simulink model "MasterArbeit_EreignisgeneratorsNachTotzone"  (R2014a)
settings: Solver=ode45  StartTime=0  StopTime=25  RelTol=1e-3
StopFcn:
  | Evaluation
values from neighbouring files (symbols this model uses):
  Ereignis_Abtastzeit = 200    [DelayDensity_GeneticAlgorithm.m]
  Ereignisgenerator_Sampletime = 0.01    [DelayDensity_GeneticAlgorithm.m]
  Instanz = ResponstimeOfCase3(1:NumOfTask)/1000    [DelayDensity_FP_Simulation.m]    (also in LatenzInstanzErzeuger.m = zeros(1,Anzahl); LatenzInstanzErzeuger_Test.m = ResponstimeOfTask)
  Kd = 0.3    [DelayDensity_GeneticAlgorithm.m]
  Ki = 4    [DelayDensity_GeneticAlgorithm.m]
  Kp = 2    [DelayDensity_GeneticAlgorithm.m]
  NumOfTask = 40    [DelayDensityTestScript.m]    (also in DelayDensity_AConcrete_Generator.m = 2; DelayDensity_GeneticAlgorithm.m = 100; DelayDensity_OberschrankenTest_Script.m = 10; DelayDensity_OberschrankenTest_Script_5Tasks.m = 10)
  rho_Wert = 0.001    [DelayDensity_GeneticAlgorithm.m]
  sollwert = 15    [DelayDensityTestScript.m]    (also in DelayDensity_GeneticAlgorithm.m = 10)
  System_A = [0 1 0;0 0 1;0 -C/A -B/A]    [DelayDensity_GeneticAlgorithm.m]
  System_B = [0;0;1/A]    [DelayDensity_GeneticAlgorithm.m]
  System_S1 = [0;0;S1/A]    [DelayDensity_GeneticAlgorithm.m]
  System_S2 = [0;0;S2/A]    [DelayDensity_GeneticAlgorithm.m]
  time1 = StartTimeOfCase3(1:NumOfTask)/1000    [DelayDensity_FP_Simulation.m]    (also in LatenzInstanzErzeuger_Test.m = StartTimeOfTask)
  Totzone_Wert = 0.1    [DelayDensity_GeneticAlgorithm.m]
  Umax = 500    [DelayDensity_GeneticAlgorithm.m]
  V = -1/(System_C*inv(System_A-System_B*K)*System_B)    [DelayDensity_GeneticAlgorithm.m]
undefined symbols (not defined in the file or in its folder): K, magnitude
libraries: simulink x2
settings Model: Creator=shenc  LastModifiedBy=shenc

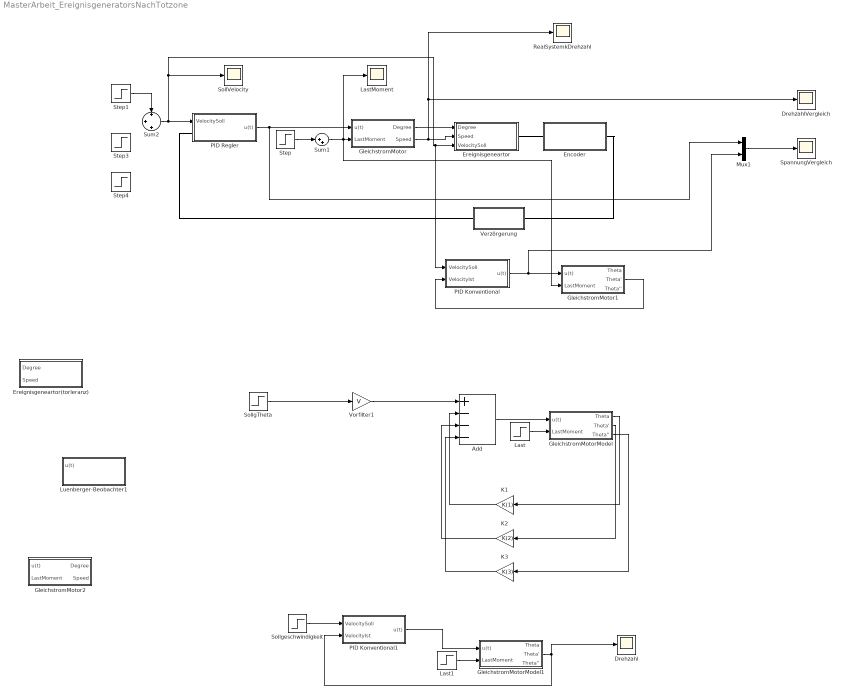
== system MasterArbeit_EreignisgeneratorsNachTotzone ==
  Add : Sum  Inputs=+---
  Drehzahl : Scope
      settings: ShowLegends=on  TimeRange=40  YMin=0  YMax=0.35  SaveName=Drehzahl1
  DrehzahlVergleich : Scope
      settings: ShowLegends=on  TimeRange=50  YMin=0  YMax=10  SaveName=Drehzahl
  Encoder : Subsystem
  Ereignisgeneartor : Subsystem
  Ereignisgeneartor(torleranz) : Subsystem
  GleichstromMotor : Subsystem
  GleichstromMotor1 : Subsystem
  GleichstromMotor2 : Subsystem
  GleichstromMotorModel : Subsystem
  GleichstromMotorModel1 : Subsystem
  K1 : Gain  Gain=K(1)
  K2 : Gain  Gain=K(2)
  K3 : Gain  Gain=K(3)
  Last : Step  Time=0  After=0  SampleTime=0
  Last1 : Step  Time=16  After=0.5  SampleTime=0
  LastMoment : Scope
      settings: ShowLegends=on  TimeRange=0.0001972721074048334  YMin=-4.75631690384965  YMax=-2.730597520382321  SaveName=ScopeData16
  Luenberger-Beobachter1 : Subsystem
  Mux1 : Mux  Inputs=2
  PID Konventional : Subsystem
  PID Konventional1 : Subsystem
  PID Regler : Subsystem
  RealSystemkDrehzahl : Scope
      settings: ShowLegends=on  TimeRange=24  YMin=9.783806343906511  YMax=15.78380634390651  SaveName=RealSystemDrehzahl
  SollVelocity : Scope
      settings: ShowLegends=on  TimeRange=0.0001972721074048334  YMin=-4.75631690384965  YMax=-2.730597520382321
  SollgTheta : Step  Time=0  After=5000  SampleTime=0
  Sollgeschwindigkeit : Step  Time=0  After=10  SampleTime=0
  SpannungVergleich : Scope
      settings: ShowLegends=on  TimeRange=0.0001972721074048334  YMin=-4.75631690384965  YMax=-2.730597520382321  SaveName=ScopeData4
  Step : Step  Time=15  After=0.3  SampleTime=0
  Step1 : Step  Time=0  After=sollwert  SampleTime=0
  Step3 : Step  Time=10  After=5  SampleTime=0
  Step4 : Step  Time=100  After=3  SampleTime=0
  Sum1 : Sum  Inputs=|++
  Sum2 : Sum  Inputs=+|+|+
  Verzörgerung : Subsystem
  Vorfilter1 : Gain  Gain=V
  wires:
  PID Regler/1(u(t)) -> Mux1/1, GleichstromMotor/1(u(t))
  Sum1/1 -> GleichstromMotor1/2(LastMoment), LastMoment/1, GleichstromMotor/2(LastMoment)
  Mux1/1 -> SpannungVergleich/1
  Sum2/1 -> PID Regler/1(VelocitySoll), PID Konventional/1(VelocitySoll), Ereignisgeneartor/3(VelocitySoll), SollVelocity/1
  Step1/1 -> Sum2/1
  GleichstromMotor/2(Speed) -> Ereignisgeneartor/2(Speed), DrehzahlVergleich/1, RealSystemkDrehzahl/1
  GleichstromMotor/1(Degree) -> Ereignisgeneartor/1(Degree)
  GleichstromMotor1/2(Theta') -> PID Konventional/2(VelocityIst)
  PID Konventional/1(u(t)) -> Mux1/2, GleichstromMotor1/1(u(t))
  Add/1 -> GleichstromMotorModel/1(u(t))
  GleichstromMotorModel/3(Theta'') -> K3/1
  K1/1 -> Add/2
  K2/1 -> Add/3
  K3/1 -> Add/4
  GleichstromMotorModel/1(Theta) -> K1/1
  GleichstromMotorModel/2(Theta') -> K2/1
  Last/1 -> GleichstromMotorModel/2(LastMoment)
  SollgTheta/1 -> Vorfilter1/1
  Vorfilter1/1 -> Add/1
  Sollgeschwindigkeit/1 -> PID Konventional1/1(VelocitySoll)
  PID Konventional1/1(u(t)) -> GleichstromMotorModel1/1(u(t))
  Last1/1 -> GleichstromMotorModel1/2(LastMoment)
  GleichstromMotorModel1/2(Theta') -> PID Konventional1/2(VelocityIst), Drehzahl/1
  Step/1 -> Sum1/1
  connections:
  Encoder/RConn1 -- Verzörgerung/LConn1
  Ereignisgeneartor/RConn1 -- Encoder/LConn1
  Verzörgerung/RConn1 -- PID Regler/LConn1

== system MasterArbeit_EreignisgeneratorsNachTotzone/Encoder ==
  Entity Sink : EntitySink
  Event-Based Entity Generator : EventBasedEntityGenerator  SignalEdgeType=Either
  Get Attribute : GetAttribute  AttributeName=Value|Speed  AttributeMissing=Error|Error  AttributeDefaultValue=1|1  AttributeTreatAsVector=1|1  AttributeSendTiming=After entity departure|After entity departure  StatNumberDeparted=on  EvaluatedDefaultAttributeValue={ [];[]}
      settings: OutputPortMap=o0,o1,o2
  Scope : Scope
      settings: SaveName=Event
  Scope1 : Scope
      settings: SaveName=Event1
  Scope2 : Scope
      settings: SaveName=Event2
  Set Attribute : SetAttribute  AttributeName=Value|Theta  AttributeFrom=Signal port|Signal port  AttributeValue=1|1  AttributeTreatAsVector=1|1  StatNumberDeparted=on  EvaluatedAttributeValue={ [];[]}
      settings: InputPortMap=u0,u1
  Degree : PMIOPort  Port=1  Side=Left
  V_Schatz : PMIOPort  Port=2  Side=Right
  wires:
  Get Attribute/3 -> Set Attribute/1, Scope2/1
  Set Attribute/1 -> Scope/1
  Get Attribute/1 -> Event-Based Entity Generator/1, Scope1/1
  Get Attribute/2 -> Set Attribute/2
  connections:
  Degree/RConn1 -- Get Attribute/LConn1
  Event-Based Entity Generator/RConn1 -- Set Attribute/LConn1
  Get Attribute/RConn1 -- Entity Sink/LConn1
  Set Attribute/RConn1 -- V_Schatz/RConn1

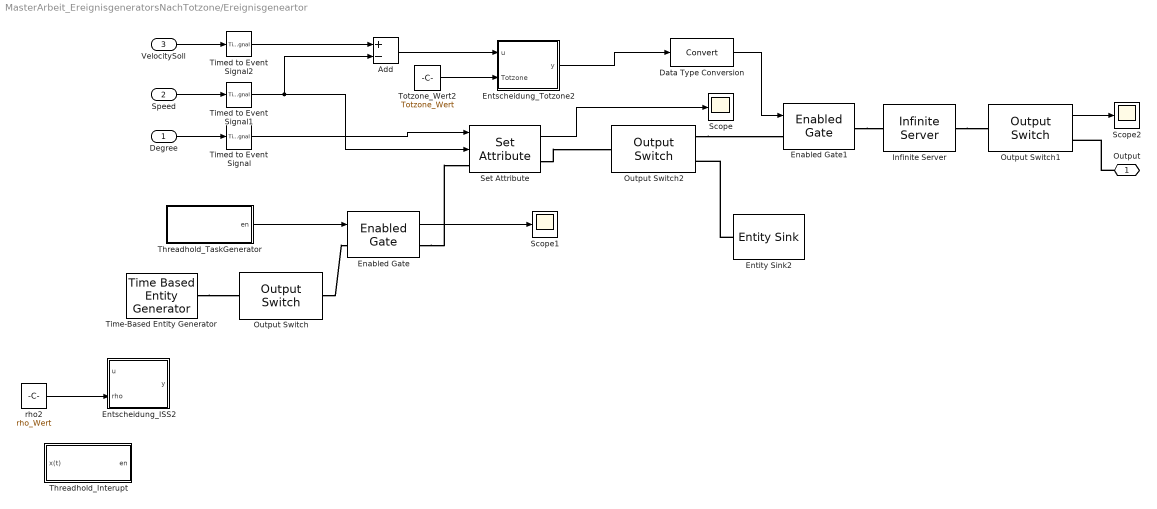
== system MasterArbeit_EreignisgeneratorsNachTotzone/Ereignisgeneartor ==
  Degree : Inport
  Speed : Inport  Port=2
  VelocitySoll : Inport  Port=3
  Add : Sum  Inputs=+-
  Data Type Conversion : DataTypeConversion
  Enabled Gate : EnabledGate  StatNumberDeparted=on
  Enabled Gate1 : EnabledGate
  Entity Sink2 : EntitySink
  Entscheidung_ISS2 : MATLAB Function  TreatAsAtomicUnit=on
  Entscheidung_Totzone2 : MATLAB Function  TreatAsAtomicUnit=on
  Infinite Server : InfiniteServer  ServiceTime=0.01
  Output Switch : OutputSwitch  NumberOutputPorts=1
  Output Switch1 : OutputSwitch  NumberOutputPorts=1  StatNumberDeparted=on
  Output Switch2 : OutputSwitch  NumberOutputPorts=2
  Scope : Scope
      settings: SaveName=ScopeData14
  Scope1 : Scope
      settings: SaveName=ScopeData19
  Scope2 : Scope
      settings: SaveName=Anzahl
  Set Attribute : SetAttribute  AttributeName=Value|Speed  AttributeFrom=Signal port|Signal port  AttributeValue=1|1  AttributeTreatAsVector=1|1  StatNumberDeparted=on  EvaluatedAttributeValue={ [];[]}
      settings: InputPortMap=u0,u1
  Threadhold_Interupt : Subsystem
  Threadhold_TaskGenerator : Subsystem
  Time-Based Entity Generator : TimeBasedEntityGenerator  Period=Ereignisgenerator_Sampletime
  Timed to Event Signal : TimedToEventSignal
  Timed to Event Signal1 : TimedToEventSignal
  Timed to Event Signal2 : TimedToEventSignal
  Totzone_Wert2 : Constant  Value=Totzone_Wert
  rho2 : Constant  Value=rho_Wert
  Output : PMIOPort  Port=1  Side=Right
  wires:
  Timed to Event Signal/1 -> Set Attribute/1
  Degree/1 -> Timed to Event Signal/1
  Speed/1 -> Timed to Event Signal1/1
  Timed to Event Signal1/1 -> Add/2, Set Attribute/2
  Data Type Conversion/1 -> Enabled Gate1/1
  VelocitySoll/1 -> Timed to Event Signal2/1
  Add/1 -> Entscheidung_Totzone2/1(u)
  Timed to Event Signal2/1 -> Add/1
  Set Attribute/1 -> Scope/1
  Enabled Gate/1 -> Scope1/1
  Output Switch1/1 -> Scope2/1
  Entscheidung_Totzone2/1(y) -> Data Type Conversion/1
  Threadhold_TaskGenerator/1(en) -> Enabled Gate/1
  rho2/1 -> Entscheidung_ISS2/2(rho)
  Totzone_Wert2/1 -> Entscheidung_Totzone2/2(Totzone)
  connections:
  Time-Based Entity Generator/RConn1 -- Output Switch/LConn1
  Output Switch/RConn1 -- Enabled Gate/LConn1
  Enabled Gate/RConn1 -- Set Attribute/LConn1
  Infinite Server/RConn1 -- Output Switch1/LConn1
  Output/RConn1 -- Output Switch1/RConn1
  Set Attribute/RConn1 -- Output Switch2/LConn1
  Entity Sink2/LConn1 -- Output Switch2/RConn2
  Output Switch2/RConn1 -- Enabled Gate1/LConn1
  Enabled Gate1/RConn1 -- Infinite Server/LConn1

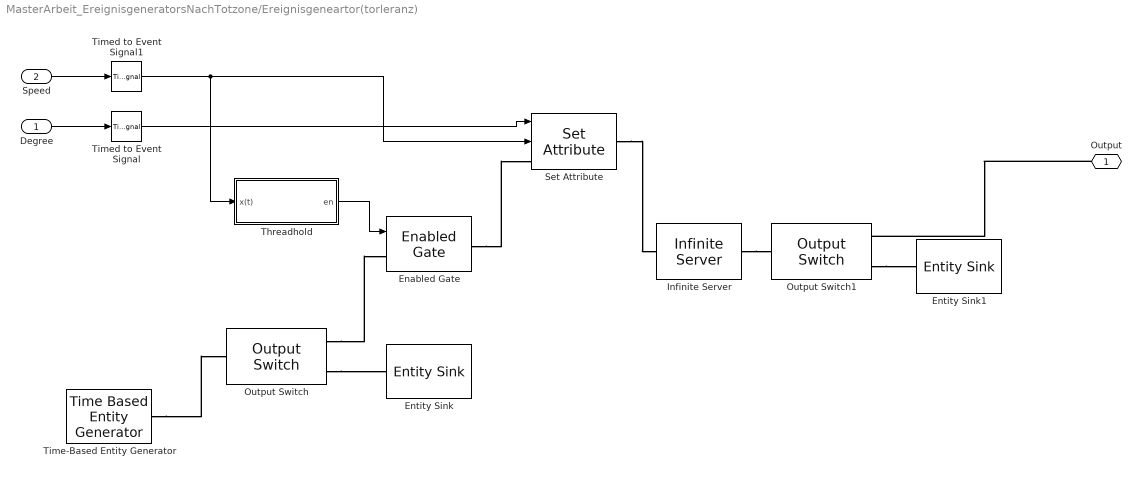
== system MasterArbeit_EreignisgeneratorsNachTotzone/Ereignisgeneartor(torleranz) ==
  Degree : Inport
  Speed : Inport  Port=2
  Enabled Gate : EnabledGate
  Entity Sink : EntitySink
  Entity Sink1 : EntitySink
  Infinite Server : InfiniteServer  ServiceTime=0.01
  Output Switch : OutputSwitch  NumberOutputPorts=2
  Output Switch1 : OutputSwitch  NumberOutputPorts=2
  Set Attribute : SetAttribute  AttributeName=Value|Speed  AttributeFrom=Signal port|Signal port  AttributeValue=1|1  AttributeTreatAsVector=1|1  EvaluatedAttributeValue={ [];[]}
      settings: InputPortMap=u0,u1
  Threadhold : Subsystem
  Time-Based Entity Generator : TimeBasedEntityGenerator  Period=Ereignisgenerator_Sampletime
  Timed to Event Signal : TimedToEventSignal
  Timed to Event Signal1 : TimedToEventSignal
  Output : PMIOPort  Port=1  Side=Right
  wires:
  Threadhold/1(en) -> Enabled Gate/1
  Timed to Event Signal/1 -> Set Attribute/1
  Degree/1 -> Timed to Event Signal/1
  Speed/1 -> Timed to Event Signal1/1
  Timed to Event Signal1/1 -> Threadhold/1(x(t)), Set Attribute/2
  connections:
  Time-Based Entity Generator/RConn1 -- Output Switch/LConn1
  Output Switch/RConn2 -- Entity Sink/LConn1
  Output Switch/RConn1 -- Enabled Gate/LConn1
  Set Attribute/RConn1 -- Infinite Server/LConn1
  Enabled Gate/RConn1 -- Set Attribute/LConn1
  Infinite Server/RConn1 -- Output Switch1/LConn1
  Output/RConn1 -- Output Switch1/RConn1
  Output Switch1/RConn2 -- Entity Sink1/LConn1

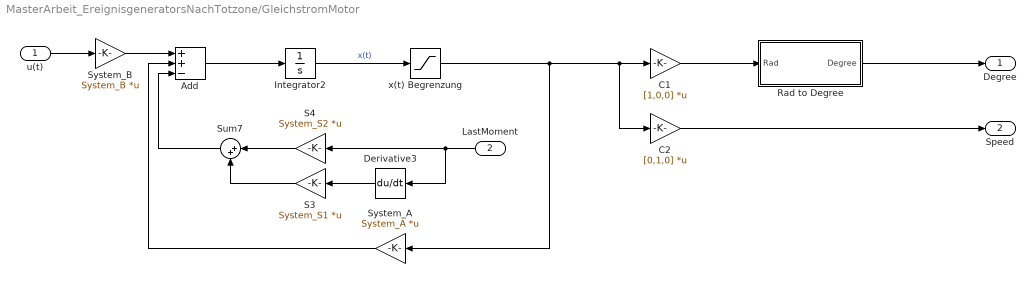
== system MasterArbeit_EreignisgeneratorsNachTotzone/GleichstromMotor ==
  u(t) : Inport
  LastMoment : Inport  Port=2
  Add : Sum  Inputs=++-
  C1 : Gain  Gain=[1,0,0]  Multiplication=Matrix(K*u)
  C2 : Gain  Gain=[0,1,0]  Multiplication=Matrix(K*u)
  Derivative3 : Derivative
  Integrator2 : Integrator
  Rad to Degree : Subsystem
  S3 : Gain  Gain=System_S1  Multiplication=Matrix(K*u)
  S4 : Gain  Gain=System_S2  Multiplication=Matrix(K*u)
  Sum7 : Sum  Inputs=|++
  System_A : Gain  Gain=System_A  Multiplication=Matrix(K*u)
  System_B : Gain  Gain=System_B  Multiplication=Matrix(K*u)
  x(t) Begrenzung : Saturate  UpperLimit=[inf,inf,20]  LowerLimit=-50
  Degree : Outport
  Speed : Outport  Port=2
  wires:
  Derivative3/1 -> S3/1
  S4/1 -> Sum7/1
  S3/1 -> Sum7/2
  u(t)/1 -> System_B/1
  C1/1 -> Rad to Degree/1(Rad)
  Integrator2/1 -> x(t) Begrenzung/1  "x(t)"
  Rad to Degree/1(Degree) -> Degree/1
  LastMoment/1 -> Derivative3/1, S4/1
  C2/1 -> Speed/1
  x(t) Begrenzung/1 -> C2/1, C1/1, System_A/1
  System_B/1 -> Add/1
  System_A/1 -> Add/2
  Sum7/1 -> Add/3
  Add/1 -> Integrator2/1

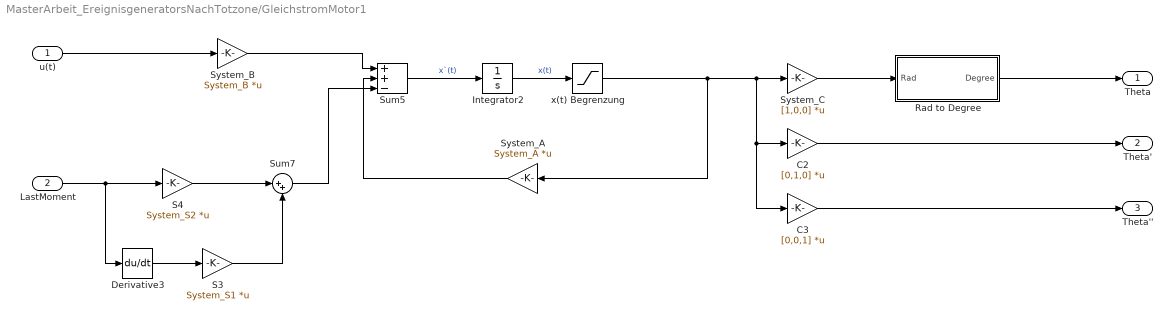
== system MasterArbeit_EreignisgeneratorsNachTotzone/GleichstromMotor1 ==
  u(t) : Inport
  LastMoment : Inport  Port=2
  C2 : Gain  Gain=[0,1,0]  Multiplication=Matrix(K*u)
  C3 : Gain  Gain=[0,0,1]  Multiplication=Matrix(K*u)
  Derivative3 : Derivative
  Integrator2 : Integrator
  Rad to Degree : Subsystem
  S3 : Gain  Gain=System_S1  Multiplication=Matrix(K*u)
  S4 : Gain  Gain=System_S2  Multiplication=Matrix(K*u)
  Sum5 : Sum  Inputs=+|+|-
  Sum7 : Sum  Inputs=|++
  System_A : Gain  Gain=System_A  Multiplication=Matrix(K*u)
  System_B : Gain  Gain=System_B  Multiplication=Matrix(K*u)
  System_C : Gain  Gain=[1,0,0]  Multiplication=Matrix(K*u)
  x(t) Begrenzung : Saturate  UpperLimit=[inf,inf,20]  LowerLimit=-50
  Theta : Outport
  Theta' : Outport  Port=2
  Theta'' : Outport  Port=3
  wires:
  Sum5/1 -> Integrator2/1  "x`(t)"
  System_A/1 -> Sum5/2
  u(t)/1 -> System_B/1
  System_B/1 -> Sum5/1
  System_C/1 -> Rad to Degree/1(Rad)
  Integrator2/1 -> x(t) Begrenzung/1  "x(t)"
  Rad to Degree/1(Degree) -> Theta/1
  C2/1 -> Theta'/1
  C3/1 -> Theta''/1
  x(t) Begrenzung/1 -> C3/1, C2/1, System_C/1, System_A/1
  LastMoment/1 -> Derivative3/1, S4/1
  S4/1 -> Sum7/1
  Derivative3/1 -> S3/1
  S3/1 -> Sum7/2
  Sum7/1 -> Sum5/3

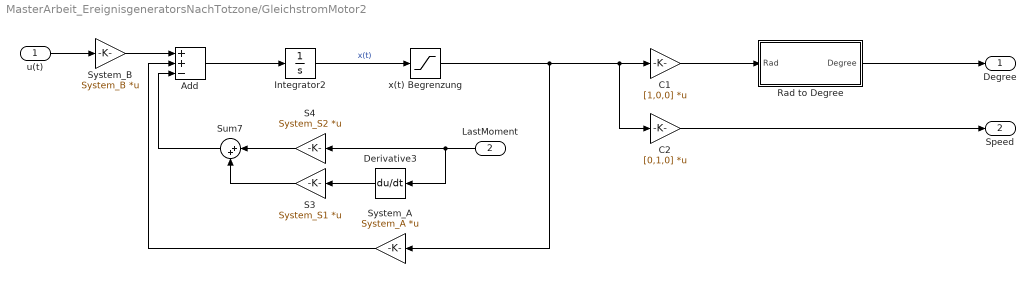
== system MasterArbeit_EreignisgeneratorsNachTotzone/GleichstromMotor2 ==
  u(t) : Inport
  LastMoment : Inport  Port=2
  Add : Sum  Inputs=++-
  C1 : Gain  Gain=[1,0,0]  Multiplication=Matrix(K*u)
  C2 : Gain  Gain=[0,1,0]  Multiplication=Matrix(K*u)
  Derivative3 : Derivative
  Integrator2 : Integrator
  Rad to Degree : Subsystem
  S3 : Gain  Gain=System_S1  Multiplication=Matrix(K*u)
  S4 : Gain  Gain=System_S2  Multiplication=Matrix(K*u)
  Sum7 : Sum  Inputs=|++
  System_A : Gain  Gain=System_A  Multiplication=Matrix(K*u)
  System_B : Gain  Gain=System_B  Multiplication=Matrix(K*u)
  x(t) Begrenzung : Saturate  UpperLimit=[inf,inf,20]  LowerLimit=-50
  Degree : Outport
  Speed : Outport  Port=2
  wires:
  Derivative3/1 -> S3/1
  S4/1 -> Sum7/1
  S3/1 -> Sum7/2
  u(t)/1 -> System_B/1
  C1/1 -> Rad to Degree/1(Rad)
  Integrator2/1 -> x(t) Begrenzung/1  "x(t)"
  Rad to Degree/1(Degree) -> Degree/1
  LastMoment/1 -> Derivative3/1, S4/1
  C2/1 -> Speed/1
  x(t) Begrenzung/1 -> C2/1, C1/1, System_A/1
  System_B/1 -> Add/1
  System_A/1 -> Add/2
  Sum7/1 -> Add/3
  Add/1 -> Integrator2/1

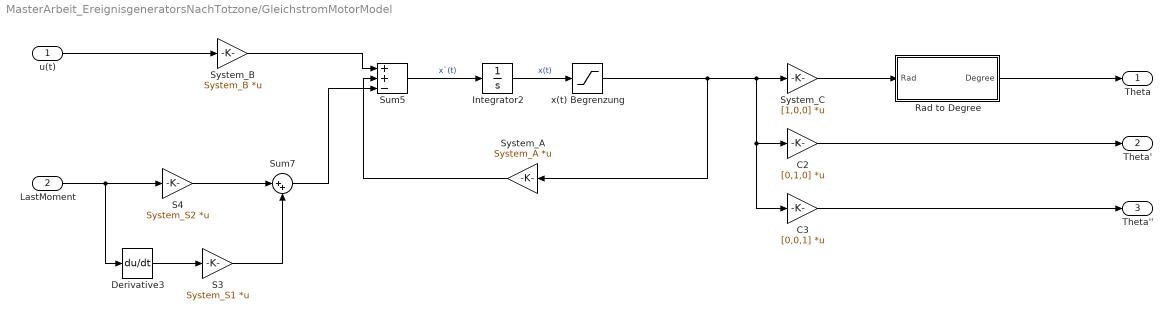
== system MasterArbeit_EreignisgeneratorsNachTotzone/GleichstromMotorModel ==
  u(t) : Inport
  LastMoment : Inport  Port=2
  C2 : Gain  Gain=[0,1,0]  Multiplication=Matrix(K*u)
  C3 : Gain  Gain=[0,0,1]  Multiplication=Matrix(K*u)
  Derivative3 : Derivative
  Integrator2 : Integrator
  Rad to Degree : Subsystem
  S3 : Gain  Gain=System_S1  Multiplication=Matrix(K*u)
  S4 : Gain  Gain=System_S2  Multiplication=Matrix(K*u)
  Sum5 : Sum  Inputs=+|+|-
  Sum7 : Sum  Inputs=|++
  System_A : Gain  Gain=System_A  Multiplication=Matrix(K*u)
  System_B : Gain  Gain=System_B  Multiplication=Matrix(K*u)
  System_C : Gain  Gain=[1,0,0]  Multiplication=Matrix(K*u)
  x(t) Begrenzung : Saturate  UpperLimit=[inf,inf,20]  LowerLimit=-50
  Theta : Outport
  Theta' : Outport  Port=2
  Theta'' : Outport  Port=3
  wires:
  Sum5/1 -> Integrator2/1  "x`(t)"
  System_A/1 -> Sum5/2
  u(t)/1 -> System_B/1
  System_B/1 -> Sum5/1
  System_C/1 -> Rad to Degree/1(Rad)
  Integrator2/1 -> x(t) Begrenzung/1  "x(t)"
  C2/1 -> Theta'/1
  C3/1 -> Theta''/1
  x(t) Begrenzung/1 -> C3/1, C2/1, System_C/1, System_A/1
  LastMoment/1 -> Derivative3/1, S4/1
  S4/1 -> Sum7/1
  Derivative3/1 -> S3/1
  S3/1 -> Sum7/2
  Sum7/1 -> Sum5/3
  Rad to Degree/1(Degree) -> Theta/1

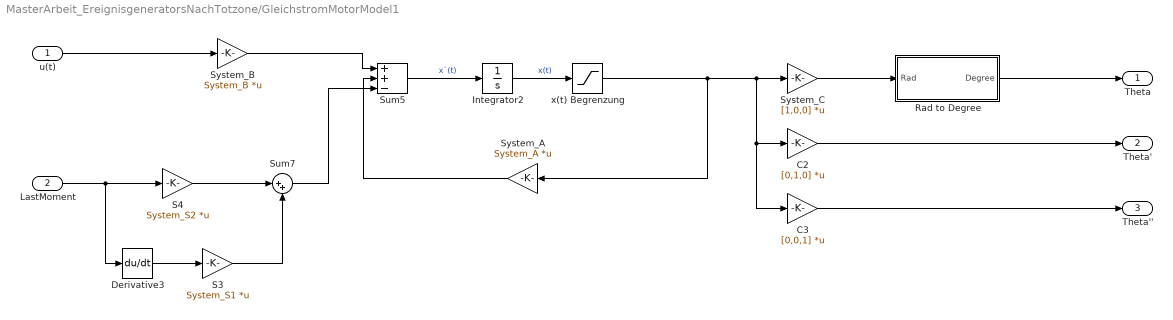
== system MasterArbeit_EreignisgeneratorsNachTotzone/GleichstromMotorModel1 ==
  u(t) : Inport
  LastMoment : Inport  Port=2
  C2 : Gain  Gain=[0,1,0]  Multiplication=Matrix(K*u)
  C3 : Gain  Gain=[0,0,1]  Multiplication=Matrix(K*u)
  Derivative3 : Derivative
  Integrator2 : Integrator
  Rad to Degree : Subsystem
  S3 : Gain  Gain=System_S1  Multiplication=Matrix(K*u)
  S4 : Gain  Gain=System_S2  Multiplication=Matrix(K*u)
  Sum5 : Sum  Inputs=+|+|-
  Sum7 : Sum  Inputs=|++
  System_A : Gain  Gain=System_A  Multiplication=Matrix(K*u)
  System_B : Gain  Gain=System_B  Multiplication=Matrix(K*u)
  System_C : Gain  Gain=[1,0,0]  Multiplication=Matrix(K*u)
  x(t) Begrenzung : Saturate  UpperLimit=[inf,inf,20]  LowerLimit=-50
  Theta : Outport
  Theta' : Outport  Port=2
  Theta'' : Outport  Port=3
  wires:
  Sum5/1 -> Integrator2/1  "x`(t)"
  System_A/1 -> Sum5/2
  u(t)/1 -> System_B/1
  System_B/1 -> Sum5/1
  System_C/1 -> Rad to Degree/1(Rad)
  Integrator2/1 -> x(t) Begrenzung/1  "x(t)"
  C2/1 -> Theta'/1
  C3/1 -> Theta''/1
  x(t) Begrenzung/1 -> C3/1, C2/1, System_C/1, System_A/1
  LastMoment/1 -> Derivative3/1, S4/1
  S4/1 -> Sum7/1
  Derivative3/1 -> S3/1
  S3/1 -> Sum7/2
  Sum7/1 -> Sum5/3
  Rad to Degree/1(Degree) -> Theta/1

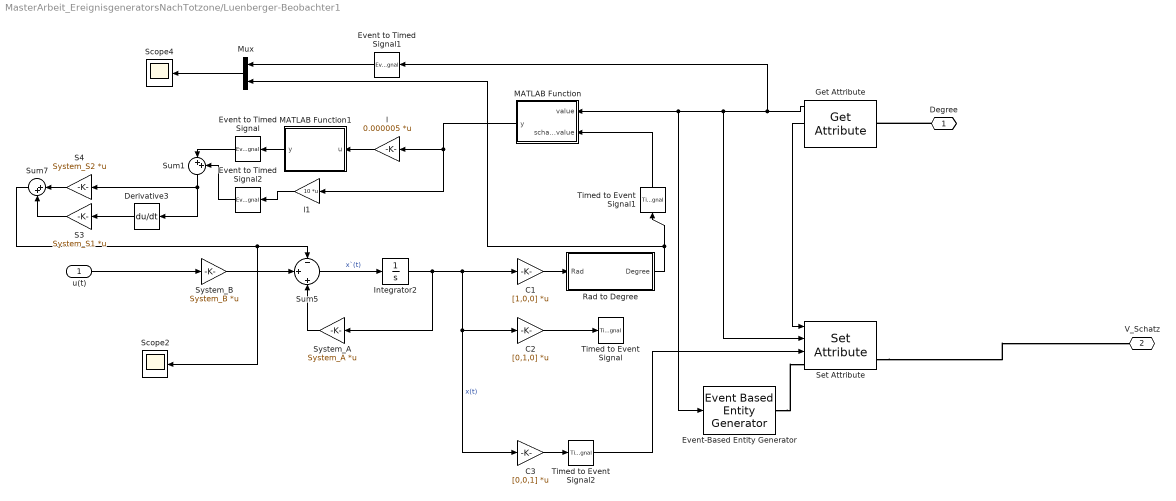
== system MasterArbeit_EreignisgeneratorsNachTotzone/Luenberger-Beobachter1 ==
  u(t) : Inport
  C1 : Gain  Gain=[1,0,0]  Multiplication=Matrix(K*u)
  C2 : Gain  Gain=[0,1,0]  Multiplication=Matrix(K*u)
  C3 : Gain  Gain=[0,0,1]  Multiplication=Matrix(K*u)
  Derivative3 : Derivative
  Event to Timed Signal : EventToTimedSignal
  Event to Timed Signal1 : EventToTimedSignal
  Event to Timed Signal2 : EventToTimedSignal
  Event-Based Entity Generator : EventBasedEntityGenerator  SignalEdgeType=Either
  Get Attribute : GetAttribute  AttributeName=Value|Speed  AttributeMissing=Error|Error  AttributeDefaultValue=1|1  AttributeTreatAsVector=1|1  AttributeSendTiming=After entity departure|After entity departure  EvaluatedDefaultAttributeValue={ [];[]}
      settings: OutputPortMap=o1,o2
  Integrator2 : Integrator
  MATLAB Function : MATLAB Function  TreatAsAtomicUnit=on
  MATLAB Function1 : MATLAB Function  TreatAsAtomicUnit=on
  Mux : Mux  Inputs=2
  Rad to Degree : Subsystem
  S3 : Gain  Gain=System_S1  Multiplication=Matrix(K*u)
  S4 : Gain  Gain=System_S2  Multiplication=Matrix(K*u)
  Scope2 : Scope
      settings: ShowLegends=on  TimeRange=10  YMin=0  YMax=275  SaveName=ScopeData15
  Scope4 : Scope
      settings: ShowLegends=on  TimeRange=10  YMin=0  YMax=275  SaveName=ScopeData13
  Set Attribute : SetAttribute  AttributeName=Value|Theta|Beschleunigung  AttributeFrom=Signal port|Signal port|Signal port  AttributeValue=1|1|1  AttributeTreatAsVector=1|1|1  StatNumberDeparted=on  EvaluatedAttributeValue={ [];[];[]}
      settings: InputPortMap=u0,u1,u2
  Sum1 : Sum  Inputs=|++
  Sum5 : Sum  Inputs=-|+|+
  Sum7 : Sum  Inputs=|++
  System_A : Gain  Gain=System_A  Multiplication=Matrix(K*u)
  System_B : Gain  Gain=System_B  Multiplication=Matrix(K*u)
  Timed to Event Signal : TimedToEventSignal
  Timed to Event Signal1 : TimedToEventSignal
  Timed to Event Signal2 : TimedToEventSignal
  l : Gain  Gain=0.000005  Multiplication=Matrix(K*u)
  l1 : Gain  Gain=10  Multiplication=Matrix(K*u)
  Degree : PMIOPort  Port=1  Side=Left
  V_Schatz : PMIOPort  Port=2  Side=Right
  wires:
  C1/1 -> Rad to Degree/1(Rad)
  Integrator2/1 -> System_A/1, C2/1, C3/1, C1/1  "x(t)"
  System_B/1 -> Sum5/2
  System_A/1 -> Sum5/3
  C3/1 -> Timed to Event Signal2/1
  Sum5/1 -> Integrator2/1  "x`(t)"
  Get Attribute/1 -> Event to Timed Signal1/1, Set Attribute/2, MATLAB Function/1(value), Event-Based Entity Generator/1
  Timed to Event Signal2/1 -> Set Attribute/3
  Mux/1 -> Scope4/1
  Rad to Degree/1(Degree) -> Mux/2, Timed to Event Signal1/1
  Timed to Event Signal1/1 -> MATLAB Function/2(schatzvalue)
  Event to Timed Signal1/1 -> Mux/1
  u(t)/1 -> System_B/1
  Derivative3/1 -> S3/1
  S4/1 -> Sum7/1
  S3/1 -> Sum7/2
  Sum7/1 -> Sum5/1, Scope2/1
  l/1 -> MATLAB Function1/1(u)
  MATLAB Function1/1(y) -> Event to Timed Signal/1
  MATLAB Function/1(y) -> l1/1, l/1
  C2/1 -> Timed to Event Signal/1
  Sum1/1 -> S4/1, Derivative3/1
  l1/1 -> Event to Timed Signal2/1
  Event to Timed Signal2/1 -> Sum1/2
  Event to Timed Signal/1 -> Sum1/1
  Get Attribute/2 -> Set Attribute/1
  connections:
  Degree/RConn1 -- Get Attribute/LConn1
  Event-Based Entity Generator/RConn1 -- Set Attribute/LConn1
  Set Attribute/RConn1 -- V_Schatz/RConn1

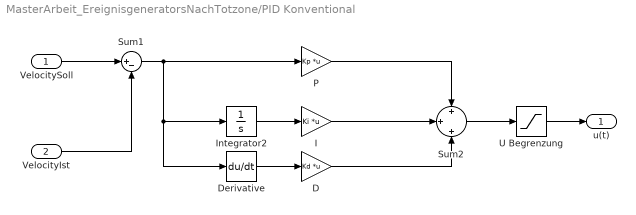
== system MasterArbeit_EreignisgeneratorsNachTotzone/PID Konventional ==
  VelocitySoll : Inport
  VelocityIst : Inport  Port=2
  D : Gain  Gain=Kd  Multiplication=Matrix(K*u)
  Derivative : Derivative
  I : Gain  Gain=Ki  Multiplication=Matrix(K*u)
  Integrator2 : Integrator
  P : Gain  Gain=Kp  Multiplication=Matrix(K*u)
  Sum1 : Sum  Inputs=|+-
  Sum2 : Sum  Inputs=+|+|+
  U Begrenzung : Saturate  UpperLimit=Umax  LowerLimit=0  ZeroCross=off
  u(t) : Outport
  wires:
  Integrator2/1 -> I/1
  Derivative/1 -> D/1
  VelocitySoll/1 -> Sum1/1
  U Begrenzung/1 -> u(t)/1
  Sum2/1 -> U Begrenzung/1
  P/1 -> Sum2/1
  Sum1/1 -> Derivative/1, Integrator2/1, P/1
  VelocityIst/1 -> Sum1/2
  I/1 -> Sum2/2
  D/1 -> Sum2/3

== system MasterArbeit_EreignisgeneratorsNachTotzone/PID Konventional1 ==
  VelocitySoll : Inport
  VelocityIst : Inport  Port=2
  D : Gain  Gain=Kd  Multiplication=Matrix(K*u)
  Derivative : Derivative
  I : Gain  Gain=Ki  Multiplication=Matrix(K*u)
  Integrator2 : Integrator
  P : Gain  Gain=Kp  Multiplication=Matrix(K*u)
  Sum1 : Sum  Inputs=|+-
  Sum2 : Sum  Inputs=+|+|+
  U Begrenzung : Saturate  UpperLimit=Umax  LowerLimit=0  ZeroCross=off
  u(t) : Outport
  wires:
  Integrator2/1 -> I/1
  Derivative/1 -> D/1
  VelocitySoll/1 -> Sum1/1
  U Begrenzung/1 -> u(t)/1
  Sum2/1 -> U Begrenzung/1
  P/1 -> Sum2/1
  Sum1/1 -> Derivative/1, Integrator2/1, P/1
  VelocityIst/1 -> Sum1/2
  I/1 -> Sum2/2
  D/1 -> Sum2/3

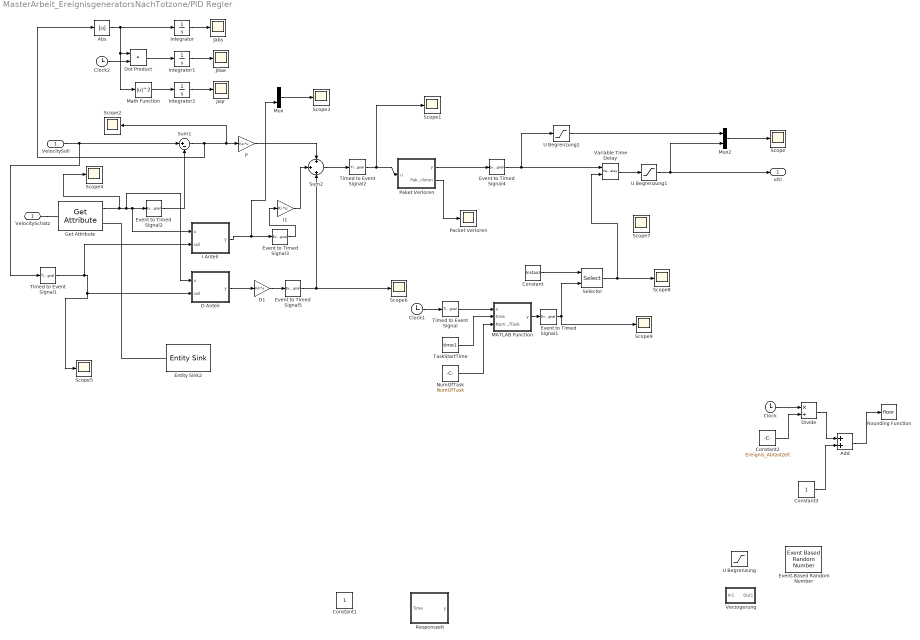
== system MasterArbeit_EreignisgeneratorsNachTotzone/PID Regler ==
  VelocitySoll : Inport
  Abs : Abs
  Add : Sum
  Clock : Clock
  Clock1 : Clock
  Clock2 : Clock
  Constant : Constant  Value=Instanz
  Constant1 : Constant
  Constant2 : Constant  Value=Ereignis_Abtastzeit
  Constant3 : Constant
  D Anteil : MATLAB Function  TreatAsAtomicUnit=on
  D1 : Gain  Gain=Kd  Multiplication=Matrix(K*u)
  Divide : Product  Inputs=*/
  Dot Product : DotProduct  InputSameDT=on  OutDataTypeStr=Inherit: Inherit via internal rule
  Entity Sink2 : EntitySink
  Event to Timed Signal{1..5} (5 alike) : EventToTimedSignal
  Event-Based Random Number : EventBasedRandomNumber  Distribution=Uniform  minUnif=0.1  maxUnif=0.5  stdNorm=0.1  meanPoiss=0.5  Seed=20361
  Get Attribute : GetAttribute  AttributeName=Value  EvaluatedDefaultAttributeValue={ []}
      settings: OutputPortMap=o1
  I Anteil : MATLAB Function  TreatAsAtomicUnit=on
  I1 : Gain  Gain=Ki  Multiplication=Matrix(K*u)
  Integrator : Integrator
  Integrator1 : Integrator
  Integrator2 : Integrator
  Jabs : Scope
      settings: TimeRange=10  YMin=7.5  YMax=10  SaveName=Jabs
  Jitae : Scope
      settings: TimeRange=10  YMin=7.5  YMax=10  SaveName=Jitae
  Jsqr : Scope
      settings: TimeRange=10  YMin=7.5  YMax=10  SaveName=Jsqr
  MATLAB Function : MATLAB Function  TreatAsAtomicUnit=on
  Math Function : Math  Operator=magnitude^2  SaturateOnIntegerOverflow=on
  Mux : Mux  Inputs=2
  Mux2 : Mux  Inputs=2
  NumOfTask : Constant  Value=NumOfTask
  P : Gain  Gain=Kp  Multiplication=Matrix(K*u)
  Packet Verloren : Scope
      settings: SaveName=ScopeData7
  Paket Verloren : MATLAB Function  TreatAsAtomicUnit=on
  Responszeit : MATLAB Function  TreatAsAtomicUnit=on
  Rounding Function : Rounding
  Scope{,1..9} (10 alike) : Scope
      Scope settings: ShowLegends=on  TimeRange=4.131253362022592  YMin=142.558  YMax=157.564
      Scope1 settings: TimeRange=80  YMin=2  YMax=22  SaveName=ScopeData6
      Scope2 settings: SaveName=ScopeData9
      Scope3 settings: TimeRange=10  YMin=7.5  YMax=10  SaveName=ScopeData10
      Scope4 settings: TimeRange=10  YMin=7.5  YMax=10  SaveName=ScopeData12
      Scope5 settings: TimeRange=10  YMin=7.5  YMax=10  SaveName=ScopeData5
      Scope6 settings: ShowLegends=on  TimeRange=10  YMin=7.5  YMax=10  SaveName=ScopeData8
      Scope7 settings: SaveName=Delay
      Scope8 settings: ShowLegends=on  TimeRange=450  YMin=2  YMax=6  SaveName=ScopeData17
      Scope9 settings: ShowLegends=on  TimeRange=4.131253362022592  YMin=13.68574199806013  YMax=16.67313288069835  SaveName=ScopeData20
  Selector : Selector  InputPortWidth=NumOfTask  IndexOptions=Index vector (port)  Indices=[1 3]
  Sum1 : Sum  Inputs=|+-
  Sum2 : Sum  Inputs=+|+|+
  TaskStartTime : Constant  Value=time1
  Timed to Event Signal : TimedToEventSignal
  Timed to Event Signal1 : TimedToEventSignal
  Timed to Event Signal2 : TimedToEventSignal
  U Begrenzung : Saturate  UpperLimit=Umax  LowerLimit=0  ZeroCross=off
  U Begrenzung1 : Saturate  UpperLimit=Umax  LowerLimit=0  ZeroCross=off
  U Begrenzung2 : Saturate  UpperLimit=Umax  LowerLimit=0  ZeroCross=off
  Variable Time Delay : VariableTransportDelay  VariableDelayType=Variable transport delay  MaximumDelay=20
  Verzogerung : Subsystem
  VelocitySchatz : PMIOPort  Port=1  Side=Left
  u(t) : Outport
  wires:
  VelocitySoll/1 -> Timed to Event Signal1/1, Sum1/1
  Sum2/1 -> Timed to Event Signal2/1
  Get Attribute/1 -> Scope4/1, D Anteil/1(u), I Anteil/1(u), Event to Timed Signal2/1
  Event to Timed Signal2/1 -> Sum1/2
  P/1 -> Sum2/1
  Sum1/1 -> Abs/1, Scope2/1, P/1
  I Anteil/1(y) -> Mux/2, Event to Timed Signal3/1
  Event to Timed Signal3/1 -> I1/1
  Mux/1 -> Scope3/1
  Timed to Event Signal2/1 -> Scope1/1, Paket Verloren/1(u)
  Paket Verloren/1(y) -> Event to Timed Signal4/1
  Event to Timed Signal4/1 -> Variable Time Delay/1, U Begrenzung2/1
  Paket Verloren/2(PaketVerloren) -> Packet Verloren/1
  Mux2/1 -> Scope/1
  D Anteil/1(y) -> D1/1
  D1/1 -> Event to Timed Signal5/1
  Event to Timed Signal5/1 -> Scope6/1, Sum2/3
  Timed to Event Signal1/1 -> I Anteil/2(soll), D Anteil/2(soll), Scope5/1
  I1/1 -> Sum2/2
  U Begrenzung2/1 -> Mux2/1
  Variable Time Delay/1 -> U Begrenzung1/1
  Selector/1 -> Variable Time Delay/2, Scope8/1
  Constant/1 -> Selector/1
  Clock/1 -> Divide/1
  Constant2/1 -> Divide/2
  Divide/1 -> Add/1
  Constant3/1 -> Add/2
  Add/1 -> Rounding Function/1
  Clock1/1 -> Timed to Event Signal/1
  Timed to Event Signal/1 -> MATLAB Function/1(u)
  TaskStartTime/1 -> MATLAB Function/2(time)
  MATLAB Function/1(y) -> Event to Timed Signal1/1
  Event to Timed Signal1/1 -> Selector/2, Scope9/1
  Abs/1 -> Math Function/1, Dot Product/1, Integrator/1
  Integrator/1 -> Jabs/1
  Clock2/1 -> Dot Product/2
  Dot Product/1 -> Integrator1/1
  Integrator1/1 -> Jitae/1
  Math Function/1 -> Integrator2/1
  Integrator2/1 -> Jsqr/1
  NumOfTask/1 -> MATLAB Function/3(NumOfTask)
  U Begrenzung1/1 -> Mux2/2, u(t)/1
  connections:
  VelocitySchatz/RConn1 -- Get Attribute/LConn1
  Entity Sink2/LConn1 -- Get Attribute/RConn1

== system MasterArbeit_EreignisgeneratorsNachTotzone/Verzörgerung ==
  Event-Based Random Number : EventBasedRandomNumber  Distribution=Uniform  maxUnif=0  stdNorm=0.1  Seed=34567
  N-Server : NServer  NumberOfServers=1  ServiceTimeFrom=Signal port t
  Input : PMIOPort  Port=1  Side=Left
  V_Schatz : PMIOPort  Port=2  Side=Right
  wires:
  Event-Based Random Number/1 -> N-Server/1
  connections:
  Input/RConn1 -- N-Server/LConn1
  N-Server/RConn1 -- V_Schatz/RConn1

== system MasterArbeit_EreignisgeneratorsNachTotzone/Ereignisgeneartor/Threadhold_Interupt ==
  x(t) : Inport
  Compare To Constant : simulink/Logic and Bit Operations/Compare To Constant  relop===  const=0  OutDataTypeStr=boolean
  Constant : Constant  Value=180
  Data Type Conversion : DataTypeConversion
  Math Function : Math  Operator=mod  OutputSignalType=real  SaturateOnIntegerOverflow=on
  Zustand : Scope
      settings: TimeRange=24.40000000000001  YMin=-4.330708661417323  YMax=-0.3307086614173231  SaveName=ScopeData2
  Zustand1 : Scope
      settings: TimeRange=24.40000000000001  YMin=-4.330708661417323  YMax=-0.3307086614173231  SaveName=ScopeData25
  en : Outport
  wires:
  x(t)/1 -> Math Function/1
  Constant/1 -> Math Function/2
  Math Function/1 -> Zustand1/1, Compare To Constant/1
  Compare To Constant/1 -> Data Type Conversion/1, Zustand/1
  Data Type Conversion/1 -> en/1

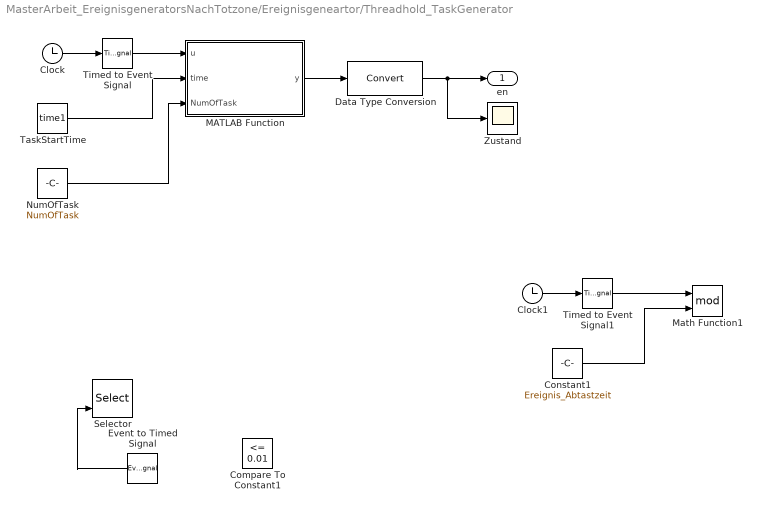
== system MasterArbeit_EreignisgeneratorsNachTotzone/Ereignisgeneartor/Threadhold_TaskGenerator ==
  Clock : Clock
  Clock1 : Clock
  Compare To Constant1 : simulink/Logic and Bit Operations/Compare To Constant  relop=<=  const=0.01  OutDataTypeStr=boolean
  Constant1 : Constant  Value=Ereignis_Abtastzeit
  Data Type Conversion : DataTypeConversion
  Event to Timed Signal : EventToTimedSignal
  MATLAB Function : MATLAB Function  TreatAsAtomicUnit=on
  Math Function1 : Math  Operator=mod  SaturateOnIntegerOverflow=on
  NumOfTask : Constant  Value=NumOfTask
  Selector : Selector  InputPortWidth=20  IndexOptions=Index vector (port)  Indices=[1 3]
  TaskStartTime : Constant  Value=time1
  Timed to Event Signal : TimedToEventSignal
  Timed to Event Signal1 : TimedToEventSignal
  Zustand : Scope
      settings: SaveName=ScopeData2
  en : Outport
  wires:
  MATLAB Function/1(y) -> Data Type Conversion/1
  Data Type Conversion/1 -> en/1, Zustand/1
  Clock/1 -> Timed to Event Signal/1
  Timed to Event Signal/1 -> MATLAB Function/1(u)
  Constant1/1 -> Math Function1/2
  Clock1/1 -> Timed to Event Signal1/1
  Timed to Event Signal1/1 -> Math Function1/1
  Event to Timed Signal/1 -> Selector/2
  TaskStartTime/1 -> MATLAB Function/2(time)
  NumOfTask/1 -> MATLAB Function/3(NumOfTask)

== system MasterArbeit_EreignisgeneratorsNachTotzone/Ereignisgeneartor(torleranz)/Threadhold ==
  x(t) : Inport
  Abs : MATLAB Function  TreatAsAtomicUnit=on
  Constant : Constant  Value=2
  Data Type Conversion : DataTypeConversion
  Subtract : Sum  Inputs=+-
  Zustand : Scope
      settings: YMin=0.95  YMax=1.05  SaveName=ScopeData2
  Zustand1 : Scope
      settings: YMin=360  YMax=360  SaveName=ScopeData3
  en : Outport
  wires:
  x(t)/1 -> Subtract/1
  Constant/1 -> Subtract/2
  Data Type Conversion/1 -> en/1
  Abs/1(y) -> Zustand/1, Data Type Conversion/1
  Subtract/1 -> Zustand1/1, Abs/1(u)

== system MasterArbeit_EreignisgeneratorsNachTotzone/GleichstromMotor/Rad to Degree ==
  Rad : Inport
  Divide : Product  Inputs=*/
  Gain : Gain  Gain=180
  Pi : Constant  Value=pi
  Rounding Function1 : Rounding
  U Begrenzung : Saturate  UpperLimit=inf  LowerLimit=1  ZeroCross=off
  Degree : Outport
  wires:
  Rad/1 -> Divide/1
  Pi/1 -> Divide/2
  Divide/1 -> Gain/1
  Rounding Function1/1 -> U Begrenzung/1
  Gain/1 -> Rounding Function1/1
  U Begrenzung/1 -> Degree/1

== system MasterArbeit_EreignisgeneratorsNachTotzone/GleichstromMotor1/Rad to Degree ==
  Rad : Inport
  Divide : Product  Inputs=*/
  Gain : Gain  Gain=180
  Pi : Constant  Value=pi
  Degree : Outport
  wires:
  Rad/1 -> Divide/1
  Pi/1 -> Divide/2
  Divide/1 -> Gain/1
  Gain/1 -> Degree/1

== system MasterArbeit_EreignisgeneratorsNachTotzone/GleichstromMotor2/Rad to Degree ==
  Rad : Inport
  Divide : Product  Inputs=*/
  Gain : Gain  Gain=180
  Pi : Constant  Value=pi
  Rounding Function1 : Rounding
  U Begrenzung : Saturate  UpperLimit=inf  LowerLimit=1  ZeroCross=off
  Degree : Outport
  wires:
  Rad/1 -> Divide/1
  Pi/1 -> Divide/2
  Divide/1 -> Gain/1
  Rounding Function1/1 -> U Begrenzung/1
  Gain/1 -> Rounding Function1/1
  U Begrenzung/1 -> Degree/1

== system MasterArbeit_EreignisgeneratorsNachTotzone/GleichstromMotorModel/Rad to Degree ==
  Rad : Inport
  Divide : Product  Inputs=*/
  Gain : Gain  Gain=180
  Pi : Constant  Value=pi
  Degree : Outport
  wires:
  Rad/1 -> Divide/1
  Pi/1 -> Divide/2
  Divide/1 -> Gain/1
  Gain/1 -> Degree/1

== system MasterArbeit_EreignisgeneratorsNachTotzone/GleichstromMotorModel1/Rad to Degree ==
  Rad : Inport
  Divide : Product  Inputs=*/
  Gain : Gain  Gain=180
  Pi : Constant  Value=pi
  Degree : Outport
  wires:
  Rad/1 -> Divide/1
  Pi/1 -> Divide/2
  Divide/1 -> Gain/1
  Gain/1 -> Degree/1

== system MasterArbeit_EreignisgeneratorsNachTotzone/Luenberger-Beobachter1/Rad to Degree ==
  Rad : Inport
  Divide : Product  Inputs=*/
  Gain : Gain  Gain=180
  Pi : Constant  Value=pi
  Degree : Outport
  wires:
  Rad/1 -> Divide/1
  Pi/1 -> Divide/2
  Divide/1 -> Gain/1
  Gain/1 -> Degree/1

== system MasterArbeit_EreignisgeneratorsNachTotzone/PID Regler/Verzogerung ==
  In1 : Inport
  Entity Sink : EntitySink
  Event to Timed Signal : EventToTimedSignal
  Event-Based Random Number : EventBasedRandomNumber  Distribution=Uniform  minUnif=0.1  maxUnif=0.5  stdNorm=0.1  meanPoiss=0.5  Seed=20361
  Get Attribute : GetAttribute  AttributeName=Value  EvaluatedDefaultAttributeValue={ []}
      settings: OutputPortMap=o1
  N-Server : NServer  NumberOfServers=10  ServiceTimeFrom=Signal port t  StatNumberDeparted=on
  Set Attribute : SetAttribute  AttributeName=Value  AttributeFrom=Signal port  EvaluatedAttributeValue={ []}
  Time-Based Entity Generator : TimeBasedEntityGenerator  GenerateEntityAtSimulationStart=off
  Timed to Event Signal : TimedToEventSignal
  Out1 : Outport
  wires:
  In1/1 -> Timed to Event Signal/1
  Event-Based Random Number/1 -> N-Server/1
  Get Attribute/1 -> Event to Timed Signal/1
  Event to Timed Signal/1 -> Out1/1
  Timed to Event Signal/1 -> Set Attribute/1
  connections:
  Get Attribute/RConn1 -- Entity Sink/LConn1
  Time-Based Entity Generator/RConn1 -- Set Attribute/LConn1
  N-Server/LConn1 -- Set Attribute/RConn1
  N-Server/RConn1 -- Get Attribute/LConn1

== matlab function MasterArbeit_EreignisgeneratorsNachTotzone/PID Regler/Paket Verloren ==
  data: u input; y output; PaketVerloren output
function [y,PaketVerloren] = fcn(u)
%#codegen
persistent u_old;
persistent PV;
persistent PV_Wert;
persistent PV_U;
x = rand;
if isempty(u_old)
    u_old = 0;% sum
    PV = 0;
    PV_Wert=0;
    PV_U=0;
end
if(u~=u_old)
    if(x>=0)
        if(u~=PV_U)
        y=u;
        u_old=u;
        else
        y=u_old;
        end
    else
        y=u_old;
        if(PV_Wert~=u_old)
        PV=PV+1;
        PV_Wert=u_old;
        PV_U=u;
        end
        
    end
    
else
   y=u_old;
end
PaketVerloren=PV;

== matlab function MasterArbeit_EreignisgeneratorsNachTotzone/PID Regler/I Anteil ==
  data: u input; y output; soll input
function y = fcn(u,soll)
%#codegen
persistent u_old;
persistent sum;
if isempty(sum)
    sum = 0;% sum
    u_old = 0;
end
if(u_old~=u)
    sum=sum+(soll-u);
    u_old=u;
end
y = sum;

== matlab function MasterArbeit_EreignisgeneratorsNachTotzone/PID Regler/D Anteil ==
  data: u input; y output; soll input
function y = fcn(u,soll)
%#codegen
persistent k;
persistent u_alt;
persistent num1;
if isempty(k)
    k = 0;% sum
    num1=0;
    u_alt=0;
end
if(u~=u_alt)
    if(k==0)
        num1=u-soll;
        k=k+1;
        y=0;
    else
        y=(u-soll)-num1;
        num1=u-soll;
    end
else
    y=u-soll;
end

== matlab function MasterArbeit_EreignisgeneratorsNachTotzone/Luenberger-Beobachter1/MATLAB Function ==
  data: value input; y output; schatzvalue input
function y = fcn(value,schatzvalue)
%#codegen
persistent value_old;
if isempty(value_old)
    value_old = 1; % sum
end
if(value_old==value)
    y=0;
else
    y=schatzvalue-value;
    %schatzvalue-value
    value_old=value;
end

== matlab function MasterArbeit_EreignisgeneratorsNachTotzone/Luenberger-Beobachter1/MATLAB Function1 ==
  data: u input; y output
function y = fcn(u)
%#codegen
persistent sum1;
if isempty(sum1)
    sum1 = 0; % sum
end
sum1=sum1+u;
y = sum1;

== matlab function MasterArbeit_EreignisgeneratorsNachTotzone/Ereignisgeneartor(torleranz)/Threadhold/Abs ==
  data: u input; y output
function y = fcn(u)
%#codegen
if abs(u)>0.05
    y=1;
else
    y=0;
end

== matlab function MasterArbeit_EreignisgeneratorsNachTotzone/PID Regler/Responszeit ==
  data: Time input; y output
function y = fcn(Time)
%#codegen
%global Ereignis_Abtastzeit
persistent index;
if isempty(index)
    index=0;
end
if(mod(Time,20)==1)
    index=index+1;
end
y=index;
end

== matlab function MasterArbeit_EreignisgeneratorsNachTotzone/Ereignisgeneartor/Threadhold_TaskGenerator/MATLAB Function ==
  data: u input; y output; time input; NumOfTask input
function y   = fcn(u,time,NumOfTask)

persistent k;
persistent index;
if isempty(k)
    k = 0;
    index = 1;
end
debug=u;
if u>time(index) && k==0 && index<=NumOfTask-1
    y=1;
    k=1;
    index=index+1;
else
    y=0;
    k=0;
end

== matlab function MasterArbeit_EreignisgeneratorsNachTotzone/PID Regler/MATLAB Function ==
  data: u input; y output; time input; NumOfTask input
function y  = fcn(u,time,NumOfTask)

persistent k;
persistent index;
if isempty(k)
    k = 0;
    index = 1;
end
if u>=time(index) && k==0 && index<=NumOfTask-1
    k=1;
    index=index+1;
    y=index-1;
else
    y=index-1;
    k=0;
end

== matlab function MasterArbeit_EreignisgeneratorsNachTotzone/Ereignisgeneartor/Entscheidung_Totzone2 ==
  data: u input; y output; Totzone input
function y = fcn(u,Totzone)
%#codegen
if abs(u)>Totzone
    y=1;
else
    y=0;
end

== matlab function MasterArbeit_EreignisgeneratorsNachTotzone/Ereignisgeneartor/Entscheidung_ISS2 ==
  data: u input; y output; rho input
function y = fcn(u,rho)
persistent abweichung_alt;
if isempty(abweichung_alt)
    k = 0;
    abweichung_alt = 0;
end

if abs(u-abweichung_alt)>rho*abs(u)
    y=1;
    abweichung_alt=u;
else
    y=0;
end
end
